simulink subsystem "PieroHFModelz"  (R2023b)
settings: Solver=VariableStepAuto  StartTime=0.0  StopTime=10.0  RelTol=1e-3
settings Model: Creator=Hajar  LastModifiedBy=Hajar

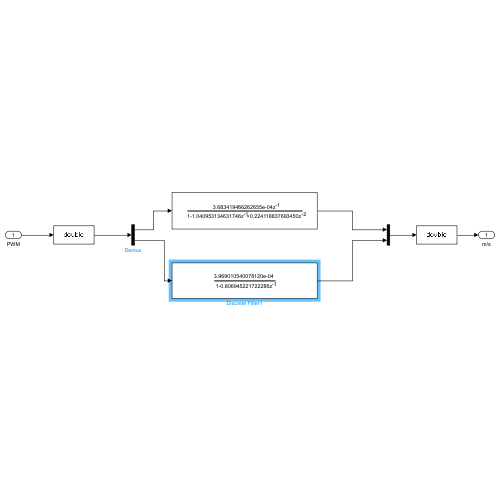
[thumbnail: Simulink's stored preview of the top-level diagram]
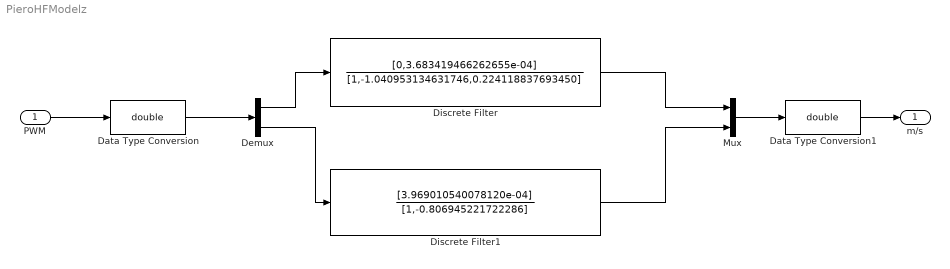
== system PieroHFModelz ==
  PWM : Inport
  Data Type Conversion : DataTypeConversion  OutDataTypeStr=double  SaturateOnIntegerOverflow=off  RndMeth=Floor
  Data Type Conversion1 : DataTypeConversion  OutDataTypeStr=double  SaturateOnIntegerOverflow=off  RndMeth=Floor
  Demux : Demux  Outputs=2
  Discrete Filter : DiscreteFilter  Numerator=[0,3.683419466262655e-04]  Denominator=[1,-1.040953134631746,0.224118837693450]
  Discrete Filter1 : DiscreteFilter  Numerator=[3.969010540078120e-04]  Denominator=[1,-0.806945221722286]
  Mux : Mux  Inputs=2
  m/s : Outport
  wires:
  Demux/1 -> Discrete Filter/1
  Demux/2 -> Discrete Filter1/1
  Discrete Filter/1 -> Mux/1
  Discrete Filter1/1 -> Mux/2
  PWM/1 -> Data Type Conversion/1
  Mux/1 -> Data Type Conversion1/1
  Data Type Conversion/1 -> Demux/1
  Data Type Conversion1/1 -> m/s/1
